simulink model "IEEE14_case"  (R2024b)
settings: Solver=FixedStepAuto  StartTime=0  StopTime=2  FixedStep=1e-7  RelTol=1e-3
values from neighbouring files (symbols this model uses):
  GFL_15_Bva = 0.009    [IEEE14_parameters.m]
  GFL_15_C_bus_pu = 7.179419    [IEEE14_parameters.m]
  GFL_15_f0 = 60    [IEEE14_parameters.m]
  GFL_15_I_id = 691.26967    [IEEE14_parameters.m]
  GFL_15_I_iq = 691.26967    [IEEE14_parameters.m]
  GFL_15_I_od = 45.2207    [IEEE14_parameters.m]
  GFL_15_I_oq = 45.2207    [IEEE14_parameters.m]
  GFL_15_I_pll = 0.78    [IEEE14_parameters.m]
  GFL_15_Kdi = 0.09    [IEEE14_parameters.m]
  GFL_15_Kdo = 0.9    [IEEE14_parameters.m]
  GFL_15_Kqi = 0.09    [IEEE14_parameters.m]
  GFL_15_Kqo = 0.9    [IEEE14_parameters.m]
  GFL_15_Lg_pu = 0.631447    [IEEE14_parameters.m]
  GFL_15_mode = 1    [IEEE14_parameters.m]
  GFL_15_P_id = 3.7166    [IEEE14_parameters.m]
  GFL_15_P_iq = 3.7166    [IEEE14_parameters.m]
  GFL_15_P_od = 0.4798    [IEEE14_parameters.m]
  GFL_15_P_oq = 0.4798    [IEEE14_parameters.m]
  GFL_15_P_pll = 290.42    [IEEE14_parameters.m]
  GFL_15_Qe_ref = 0.2    [IEEE14_parameters.m]
  GFL_15_Rg_pu = 0.024016    [IEEE14_parameters.m]
  GFL_15_Sbase = 1.000000e+4    (= 10000)    [IEEE14_parameters.m]
  GFL_15_Tdi = 0.01    [IEEE14_parameters.m]
  GFL_15_Tdo = 0.2    [IEEE14_parameters.m]
  GFL_15_Tqi = 0.01    [IEEE14_parameters.m]
  GFL_15_Tqo = 0.2    [IEEE14_parameters.m]
  GFL_15_Vbase = 380    [IEEE14_parameters.m]
  GFL_15_Vdc_ref = 1.011475    [IEEE14_parameters.m]
  GFL_15_Vdcbase = 700    [IEEE14_parameters.m]
  GFL_15_vq_ref = 0    [IEEE14_parameters.m]
  GFL_16_Bva = 0.002    [IEEE14_parameters.m]
  GFL_16_C_bus_pu = 7.179419    [IEEE14_parameters.m]
  GFL_16_f0 = 60    [IEEE14_parameters.m]
  GFL_16_I_id = 691.26967    [IEEE14_parameters.m]
  GFL_16_I_iq = 691.26967    [IEEE14_parameters.m]
  GFL_16_I_od = 45.2207    [IEEE14_parameters.m]
  GFL_16_I_oq = 45.2207    [IEEE14_parameters.m]
  GFL_16_I_pll = 0.78    [IEEE14_parameters.m]
  GFL_16_Kdi = 0.05    [IEEE14_parameters.m]
  GFL_16_Kdo = 0.5    [IEEE14_parameters.m]
  GFL_16_Kqi = 0.05    [IEEE14_parameters.m]
  GFL_16_Kqo = 0.5    [IEEE14_parameters.m]
  GFL_16_Lg_pu = 0.631447    [IEEE14_parameters.m]
  GFL_16_mode = 1    [IEEE14_parameters.m]
  GFL_16_P_id = 3.7166    [IEEE14_parameters.m]
  GFL_16_P_iq = 3.7166    [IEEE14_parameters.m]
  GFL_16_P_od = 0.4798    [IEEE14_parameters.m]
  GFL_16_P_oq = 0.4798    [IEEE14_parameters.m]
  GFL_16_P_pll = 290.42    [IEEE14_parameters.m]
  GFL_16_Qe_ref = 0.2    [IEEE14_parameters.m]
  GFL_16_Rg_pu = 0.024016    [IEEE14_parameters.m]
  GFL_16_Sbase = 1.000000e+4    (= 10000)    [IEEE14_parameters.m]
  GFL_16_Tdi = 0.01    [IEEE14_parameters.m]
  GFL_16_Tdo = 0.2    [IEEE14_parameters.m]
  GFL_16_Tqi = 0.01    [IEEE14_parameters.m]
  GFL_16_Tqo = 0.2    [IEEE14_parameters.m]
  GFL_16_Vbase = 380    [IEEE14_parameters.m]
  GFL_16_Vdc_ref = 1.01144    [IEEE14_parameters.m]
  GFL_16_Vdcbase = 700    [IEEE14_parameters.m]
  GFL_16_vq_ref = 0    [IEEE14_parameters.m]
  GFL_17_Bva = 0.002    [IEEE14_parameters.m]
  GFL_17_C_bus_pu = 7.179419    [IEEE14_parameters.m]
  GFL_17_f0 = 60    [IEEE14_parameters.m]
  GFL_17_I_id = 691.26967    [IEEE14_parameters.m]
  GFL_17_I_iq = 691.26967    [IEEE14_parameters.m]
  GFL_17_I_od = 45.2207    [IEEE14_parameters.m]
  GFL_17_I_oq = 45.2207    [IEEE14_parameters.m]
  GFL_17_I_pll = 0.78    [IEEE14_parameters.m]
  GFL_17_Kdi = 0.05    [IEEE14_parameters.m]
  GFL_17_Kdo = 0.5    [IEEE14_parameters.m]
  GFL_17_Kqi = 0.05    [IEEE14_parameters.m]
  GFL_17_Kqo = 0.5    [IEEE14_parameters.m]
  GFL_17_Lg_pu = 0.631447    [IEEE14_parameters.m]
  GFL_17_mode = 1    [IEEE14_parameters.m]
  GFL_17_P_id = 3.7166    [IEEE14_parameters.m]
  GFL_17_P_iq = 3.7166    [IEEE14_parameters.m]
  GFL_17_P_od = 0.4798    [IEEE14_parameters.m]
  GFL_17_P_oq = 0.4798    [IEEE14_parameters.m]
  GFL_17_P_pll = 290.42    [IEEE14_parameters.m]
  GFL_17_Qe_ref = 0.2    [IEEE14_parameters.m]
  GFL_17_Rg_pu = 0.024016    [IEEE14_parameters.m]
  GFL_17_Sbase = 1.000000e+4    (= 10000)    [IEEE14_parameters.m]
  GFL_17_Tdi = 0.01    [IEEE14_parameters.m]
  GFL_17_Tdo = 0.2    [IEEE14_parameters.m]
  GFL_17_Tqi = 0.01    [IEEE14_parameters.m]
  GFL_17_Tqo = 0.2    [IEEE14_parameters.m]
  GFL_17_Vbase = 380    [IEEE14_parameters.m]
  GFL_17_Vdc_ref = 1.011632    [IEEE14_parameters.m]
  GFL_17_Vdcbase = 700    [IEEE14_parameters.m]
  GFL_17_vq_ref = 0    [IEEE14_parameters.m]
  GFL_18_Bva = 0.002    [IEEE14_parameters.m]
  GFL_18_C_bus_pu = 7.179419    [IEEE14_parameters.m]
  GFL_18_f0 = 60    [IEEE14_parameters.m]
  GFL_18_I_id = 691.26967    [IEEE14_parameters.m]
  GFL_18_I_iq = 691.26967    [IEEE14_parameters.m]
  GFL_18_I_od = 45.2207    [IEEE14_parameters.m]
  GFL_18_I_oq = 45.2207    [IEEE14_parameters.m]
  GFL_18_I_pll = 0.78    [IEEE14_parameters.m]
  GFL_18_Kdi = 0.05    [IEEE14_parameters.m]
  GFL_18_Kdo = 0.5    [IEEE14_parameters.m]
  GFL_18_Kqi = 0.05    [IEEE14_parameters.m]
  GFL_18_Kqo = 0.5    [IEEE14_parameters.m]
  GFL_18_Lg_pu = 0.631447    [IEEE14_parameters.m]
  GFL_18_mode = 1    [IEEE14_parameters.m]
  GFL_18_P_id = 3.7166    [IEEE14_parameters.m]
  GFL_18_P_iq = 3.7166    [IEEE14_parameters.m]
  GFL_18_P_od = 0.4798    [IEEE14_parameters.m]
  GFL_18_P_oq = 0.4798    [IEEE14_parameters.m]
  GFL_18_P_pll = 290.42    [IEEE14_parameters.m]
  GFL_18_Qe_ref = 0.2    [IEEE14_parameters.m]
  GFL_18_Rg_pu = 0.024016    [IEEE14_parameters.m]
  GFL_18_Sbase = 1.000000e+4    (= 10000)    [IEEE14_parameters.m]
  GFL_18_Tdi = 0.01    [IEEE14_parameters.m]
  GFL_18_Tdo = 0.2    [IEEE14_parameters.m]
  GFL_18_Tqi = 0.01    [IEEE14_parameters.m]
  GFL_18_Tqo = 0.2    [IEEE14_parameters.m]
  GFL_18_Vbase = 380    [IEEE14_parameters.m]
  GFL_18_Vdc_ref = 1.011572    [IEEE14_parameters.m]
  GFL_18_Vdcbase = 700    [IEEE14_parameters.m]
  GFL_18_vq_ref = 0    [IEEE14_parameters.m]
  ... (+180 more)
(part 11 of 25)

== system IEEE14_case/GFL_16/d_Phi_gb_GFL_16_block ==
  note: d_Phi_gb_GFL_16 in case14gfl
      | $I_{\mathrm{id}}\,\left(\mathrm{Idv}_{\mathrm{GFL},16}+\Phi _{\mathrm{ga},\mathrm{GFL},16}-i_{\mathrm{gd},\mathrm{GFL},16}+P_{\mathrm{od}}\,\left(V_{\mathrm{dc},\mathrm{GFL},16}-\mathrm{Vdcbase}\,\mathrm{Vdc}_{\mathrm{ref}}\right)-\mathrm{Bva}\,\mathrm{Vbase}\,\left(v_{d,\mathrm{GFL},16}\,\cos\left(\theta _{\mathrm{pll},\mathrm{GFL},16}\right)-v_{q,\mathrm{GFL},16}\,\sin\left(\theta _{\mathrm{pll},\mathrm{GFL},16}\right)\right)\right)$
      | Automatically generated on 2025-10-09 21:36:07 .
  Input_v_d_GFL_16_5796c : Inport
  State_theta_pll_GFL_16_9faca : Inport  Port=2
  Input_v_q_GFL_16_58470 : Inport  Port=3
  State_theta_pll_GFL_16_1f0e5 : Inport  Port=4
  State_Idv_GFL_16_00ce2 : Inport  Port=5
  State_V_dc_GFL_16_186eb : Inport  Port=6
  State_Phi_ga_GFL_16_9aa12 : Inport  Port=7
  State_i_gd_GFL_16_104f5 : Inport  Port=8
  Add_816d2 : Sum
  Add_8c69a : Sum
  Add_ee524 : Sum
  Constant_-1_c479b : Constant  Value=-1
  Constant_Bva_cc442 : Constant  Value=Bva
  Constant_I_id_7e45e : Constant  Value=I_id
  Constant_P_od_57961 : Constant  Value=P_od
  Constant_Vbase_d7372 : Constant  Value=Vbase
  Constant_Vdc_ref_5c322 : Constant  Value=Vdc_ref
  Constant_Vdcbase_67ddd : Constant  Value=Vdcbase
  MathFunc_cos_ca6bf : Trigonometry  Operator=cos
  MathFunc_sin_e0267 : Trigonometry
  Product_2926b : Product
  Product_2d34a : Product
  Product_4ef76 : Product
  Product_59aab : Product
  Product_6212c : Product
  Product_b48db : Product
  Product_c4ab1 : Product
  Product_e24fb : Product
  Subtract_1bdde : Sum  Inputs=+-
  Subtract_e3d0d : Sum  Inputs=+-
  Subtract_eb397 : Sum  Inputs=+-
  Blockout_d_Phi_gb_GFL_16_e3dc3 : Outport
  wires:
  State_theta_pll_GFL_16_9faca/1 -> MathFunc_cos_ca6bf/1
  Constant_Bva_cc442/1 -> Product_c4ab1/2
  State_theta_pll_GFL_16_1f0e5/1 -> MathFunc_sin_e0267/1
  Product_c4ab1/1 -> Product_2d34a/1
  Constant_-1_c479b/1 -> Product_c4ab1/1
  Input_v_d_GFL_16_5796c/1 -> Product_59aab/1
  MathFunc_cos_ca6bf/1 -> Product_59aab/2
  Product_b48db/1 -> Subtract_1bdde/2
  Input_v_q_GFL_16_58470/1 -> Product_b48db/1
  MathFunc_sin_e0267/1 -> Product_b48db/2
  Constant_Vbase_d7372/1 -> Product_2d34a/2
  Product_59aab/1 -> Subtract_1bdde/1
  State_Phi_ga_GFL_16_9aa12/1 -> Add_816d2/2
  Constant_Vdc_ref_5c322/1 -> Product_4ef76/1
  Constant_Vdcbase_67ddd/1 -> Product_4ef76/2
  Product_2d34a/1 -> Product_e24fb/1
  Subtract_1bdde/1 -> Product_e24fb/2
  State_i_gd_GFL_16_104f5/1 -> Subtract_e3d0d/2
  State_V_dc_GFL_16_186eb/1 -> Subtract_eb397/1
  Product_4ef76/1 -> Subtract_eb397/2
  Product_e24fb/1 -> Add_8c69a/1
  State_Idv_GFL_16_00ce2/1 -> Add_8c69a/2
  Product_2926b/1 -> Add_ee524/2
  Constant_P_od_57961/1 -> Product_2926b/1
  Subtract_eb397/1 -> Product_2926b/2
  Add_8c69a/1 -> Add_ee524/1
  Add_ee524/1 -> Add_816d2/1
  Add_816d2/1 -> Subtract_e3d0d/1
  Constant_I_id_7e45e/1 -> Product_6212c/1
  Subtract_e3d0d/1 -> Product_6212c/2
  Product_6212c/1 -> Blockout_d_Phi_gb_GFL_16_e3dc3/1

== system IEEE14_case/GFL_16/d_Phi_gc_GFL_16_block ==
  note: d_Phi_gc_GFL_16 in case14gfl
      | $-I_{\mathrm{oq}}\,\left(\mathrm{Qe}_{\mathrm{ref}}\,\mathrm{Sbase}+1.73205080756888\,\mathrm{Vbase}\,i_{\mathrm{gd},\mathrm{GFL},16}\,\left(v_{q,\mathrm{GFL},16}\,\cos\left(\theta _{\mathrm{pll},\mathrm{GFL},16}\right)+v_{d,\mathrm{GFL},16}\,\sin\left(\theta _{\mathrm{pll},\mathrm{GFL},16}\right)\right)+1.73205080756888\,\mathrm{Vbase}\,i_{\mathrm{gq},\mathrm{GFL},16}\,\left(v_{d,\mathrm{GFL},16}\,\cos\left(\theta _{\mathrm{pll},\mathrm{GFL},16}\right)-v_{q,\mathrm{GFL},16}\,\sin\left(\theta _{\mathrm{pll},\mathrm{GFL},16}\right)\right)\right)$
      | Automatically generated on 2025-10-09 21:36:09 .
  State_i_gd_GFL_16_f5bc3 : Inport
  Input_v_d_GFL_16_5298e : Inport  Port=2
  State_theta_pll_GFL_16_2a2ae : Inport  Port=3
  Input_v_q_GFL_16_b8cf3 : Inport  Port=4
  State_theta_pll_GFL_16_9a1c0 : Inport  Port=5
  State_i_gq_GFL_16_12809 : Inport  Port=6
  Input_v_d_GFL_16_c77ca : Inport  Port=7
  State_theta_pll_GFL_16_c56ef : Inport  Port=8
  Input_v_q_GFL_16_61e16 : Inport  Port=9
  State_theta_pll_GFL_16_a6854 : Inport  Port=10
  Add_9f244 : Sum
  Constant_-1_d068e : Constant  Value=-1
  Constant_1.73205080756888_1ab3f : Constant  Value=1.73205080756888
  Constant_1.73205080756888_3e260 : Constant  Value=1.73205080756888
  Constant_I_oq_16e38 : Constant  Value=I_oq
  Constant_Qe_ref_4cc63 : Constant  Value=Qe_ref
  Constant_Sbase_67194 : Constant  Value=Sbase
  Constant_Vbase_67024 : Constant  Value=Vbase
  Constant_Vbase_c2ada : Constant  Value=Vbase
  MathFunc_cos_8d063 : Trigonometry  Operator=cos
  MathFunc_cos_e387c : Trigonometry  Operator=cos
  MathFunc_sin_1c9af : Trigonometry
  MathFunc_sin_fc0e6 : Trigonometry
  Product_1eb07 : Product
  Product_2f77b : Product
  Product_396d7 : Product
  Product_4fce4 : Product
  Product_59751 : Product
  Product_6bdde : Product
  Product_70e4a : Product
  Product_73ed6 : Product
  Product_b9821 : Product
  Product_c0659 : Product
  Product_e5fa5 : Product
  Product_ed71a : Product
  Product_f25bb : Product
  Subtract_08a0b : Sum  Inputs=+-
  Subtract_bd4c9 : Sum  Inputs=+-
  Subtract_ee10c : Sum  Inputs=+-
  Blockout_d_Phi_gc_GFL_16_21552 : Outport
  wires:
  Product_c0659/1 -> Product_2f77b/1
  Constant_Vbase_c2ada/1 -> Product_4fce4/2
  State_theta_pll_GFL_16_2a2ae/1 -> MathFunc_sin_1c9af/1
  State_theta_pll_GFL_16_9a1c0/1 -> MathFunc_cos_e387c/1
  MathFunc_cos_e387c/1 -> Product_b9821/2
  Product_4fce4/1 -> Product_c0659/1
  Constant_1.73205080756888_3e260/1 -> Product_4fce4/1
  Product_e5fa5/1 -> Add_9f244/1
  Input_v_d_GFL_16_5298e/1 -> Product_e5fa5/1
  MathFunc_sin_1c9af/1 -> Product_e5fa5/2
  Product_b9821/1 -> Add_9f244/2
  Input_v_q_GFL_16_b8cf3/1 -> Product_b9821/1
  MathFunc_cos_8d063/1 -> Product_59751/2
  State_theta_pll_GFL_16_c56ef/1 -> MathFunc_cos_8d063/1
  MathFunc_sin_fc0e6/1 -> Product_f25bb/2
  State_theta_pll_GFL_16_a6854/1 -> MathFunc_sin_fc0e6/1
  Constant_-1_d068e/1 -> Product_1eb07/1
  Product_2f77b/1 -> Subtract_bd4c9/2
  Constant_Qe_ref_4cc63/1 -> Product_1eb07/2
  State_i_gd_GFL_16_f5bc3/1 -> Product_c0659/2
  Product_396d7/1 -> Product_6bdde/1
  Constant_1.73205080756888_1ab3f/1 -> Product_396d7/1
  Product_6bdde/1 -> Product_73ed6/1
  Constant_Vbase_67024/1 -> Product_396d7/2
  Product_59751/1 -> Subtract_08a0b/1
  Product_1eb07/1 -> Product_70e4a/1
  Input_v_d_GFL_16_c77ca/1 -> Product_59751/1
  Input_v_q_GFL_16_61e16/1 -> Product_f25bb/1
  Constant_Sbase_67194/1 -> Product_70e4a/2
  Add_9f244/1 -> Product_2f77b/2
  Constant_I_oq_16e38/1 -> Product_ed71a/1
  State_i_gq_GFL_16_12809/1 -> Product_6bdde/2
  Product_f25bb/1 -> Subtract_08a0b/2
  Product_70e4a/1 -> Subtract_bd4c9/1
  Subtract_08a0b/1 -> Product_73ed6/2
  Subtract_bd4c9/1 -> Subtract_ee10c/1
  Product_73ed6/1 -> Subtract_ee10c/2
  Subtract_ee10c/1 -> Product_ed71a/2
  Product_ed71a/1 -> Blockout_d_Phi_gc_GFL_16_21552/1

== system IEEE14_case/GFL_16/d_Phi_gd_GFL_16_block ==
  note: d_Phi_gd_GFL_16 in case14gfl
      | $I_{\mathrm{iq}}\,\left(\mathrm{Iqv}_{\mathrm{GFL},16}+\Phi _{\mathrm{gc},\mathrm{GFL},16}-i_{\mathrm{gq},\mathrm{GFL},16}-P_{\mathrm{oq}}\,\left(\mathrm{Qe}_{\mathrm{ref}}\,\mathrm{Sbase}+1.73205080756888\,\mathrm{Vbase}\,i_{\mathrm{gd},\mathrm{GFL},16}\,\left(v_{q,\mathrm{GFL},16}\,\cos\left(\theta _{\mathrm{pll},\mathrm{GFL},16}\right)+v_{d,\mathrm{GFL},16}\,\sin\left(\theta _{\mathrm{pll},\mathrm{GFL},16}\right)\right)+1.73205080756888\,\mathrm{Vbase}\,i_{\mathrm{gq},\mathrm{GFL},16}\,\left(v_{d,\mathrm{GFL},16}\,\cos\left(\theta _{\mathrm{pll},\mathrm{GFL},16}\right)-v_{q,\mathrm{GFL},16}\,\sin\left(\theta _{\mathrm{pll},\mathrm{GFL},16}\right)\right)\right)+\mathrm{Bva}\,\mathrm{Vbase}\,\left(v_{q,\mathrm{GFL},16}\,\cos\left(\theta _{\mathrm{pll},\mathrm{GFL},16}\right)+v_{d,\mathrm{GFL},16}\,\sin\left(\theta _{\mathrm{pll},\mathrm{GFL},16}\right)\right)\right)$
      | Automatically generated on 2025-10-09 21:36:13 .
  Input_v_d_GFL_16_9b711 : Inport
  State_theta_pll_GFL_16_648b2 : Inport  Port=2
  Input_v_q_GFL_16_c9e4f : Inport  Port=3
  State_theta_pll_GFL_16_e1421 : Inport  Port=4
  State_Iqv_GFL_16_6ee1c : Inport  Port=5
  State_i_gd_GFL_16_6aeee : Inport  Port=6
  Input_v_d_GFL_16_a7f85 : Inport  Port=7
  State_theta_pll_GFL_16_9c942 : Inport  Port=8
  Input_v_q_GFL_16_d5137 : Inport  Port=9
  State_theta_pll_GFL_16_5c378 : Inport  Port=10
  State_i_gq_GFL_16_a69ee : Inport  Port=11
  Input_v_d_GFL_16_1cbf7 : Inport  Port=12
  State_theta_pll_GFL_16_6f123 : Inport  Port=13
  Input_v_q_GFL_16_69c8c : Inport  Port=14
  State_theta_pll_GFL_16_ebd89 : Inport  Port=15
  State_Phi_gc_GFL_16_a3666 : Inport  Port=16
  State_i_gq_GFL_16_a143d : Inport  Port=17
  Add_25052 : Sum
  Add_4ccd0 : Sum
  Add_8848f : Sum
  Add_ca996 : Sum
  Add_ec70f : Sum
  Constant_-1_88cd8 : Constant  Value=-1
  Constant_1.73205080756888_3396c : Constant  Value=1.73205080756888
  Constant_1.73205080756888_d617b : Constant  Value=1.73205080756888
  Constant_Bva_7e4b7 : Constant  Value=Bva
  Constant_I_iq_112b7 : Constant  Value=I_iq
  Constant_P_oq_4cce5 : Constant  Value=P_oq
  Constant_Qe_ref_93a57 : Constant  Value=Qe_ref
  Constant_Sbase_e2cd0 : Constant  Value=Sbase
  Constant_Vbase_039f5 : Constant  Value=Vbase
  Constant_Vbase_a3316 : Constant  Value=Vbase
  Constant_Vbase_be2b5 : Constant  Value=Vbase
  MathFunc_cos_518fc : Trigonometry  Operator=cos
  MathFunc_cos_a487e : Trigonometry  Operator=cos
  MathFunc_cos_c3736 : Trigonometry  Operator=cos
  MathFunc_sin_243eb : Trigonometry
  MathFunc_sin_a3588 : Trigonometry
  MathFunc_sin_bcd20 : Trigonometry
  Product_02c56 : Product
  Product_09f61 : Product
  Product_110c1 : Product
  Product_225ea : Product
  Product_2c3a6 : Product
  Product_2e02e : Product
  Product_3a99f : Product
  Product_43745 : Product
  Product_4da1f : Product
  Product_4e7c3 : Product
  Product_795ee : Product
  Product_7b424 : Product
  Product_7dc20 : Product
  Product_a6212 : Product
  Product_aac61 : Product
  Product_bbe8c : Product
  Product_c7878 : Product
  Product_e0150 : Product
  Subtract_13f81 : Sum  Inputs=+-
  Subtract_6cb63 : Sum  Inputs=+-
  Subtract_7336c : Sum  Inputs=+-
  Subtract_acad4 : Sum  Inputs=+-
  Blockout_d_Phi_gd_GFL_16_8a731 : Outport
  wires:
  State_theta_pll_GFL_16_9c942/1 -> MathFunc_sin_243eb/1
  MathFunc_sin_243eb/1 -> Product_225ea/2
  Product_7b424/1 -> Product_43745/1
  Constant_Vbase_be2b5/1 -> Product_110c1/2
  State_theta_pll_GFL_16_5c378/1 -> MathFunc_cos_a487e/1
  Constant_1.73205080756888_3396c/1 -> Product_110c1/1
  Constant_Qe_ref_93a57/1 -> Product_a6212/2
  Input_v_d_GFL_16_a7f85/1 -> Product_225ea/1
  Input_v_q_GFL_16_d5137/1 -> Product_c7878/1
  MathFunc_cos_a487e/1 -> Product_c7878/2
  State_theta_pll_GFL_16_6f123/1 -> MathFunc_cos_c3736/1
  State_theta_pll_GFL_16_ebd89/1 -> MathFunc_sin_bcd20/1
  State_Iqv_GFL_16_6ee1c/1 -> Add_ec70f/2
  State_theta_pll_GFL_16_648b2/1 -> MathFunc_sin_a3588/1
  State_theta_pll_GFL_16_e1421/1 -> MathFunc_cos_518fc/1
  Constant_-1_88cd8/1 -> Product_a6212/1
  State_i_gd_GFL_16_6aeee/1 -> Product_7b424/2
  Product_110c1/1 -> Product_7b424/1
  Product_225ea/1 -> Add_8848f/1
  Product_3a99f/1 -> Add_ec70f/1
  Product_c7878/1 -> Add_8848f/2
  Constant_Bva_7e4b7/1 -> Product_4da1f/1
  Constant_1.73205080756888_d617b/1 -> Product_7dc20/1
  Add_ec70f/1 -> Add_4ccd0/1
  Product_7dc20/1 -> Product_2e02e/1
  Constant_Vbase_a3316/1 -> Product_7dc20/2
  Input_v_d_GFL_16_1cbf7/1 -> Product_aac61/1
  MathFunc_cos_c3736/1 -> Product_aac61/2
  Product_2c3a6/1 -> Subtract_acad4/2
  Input_v_q_GFL_16_69c8c/1 -> Product_2c3a6/1
  MathFunc_sin_bcd20/1 -> Product_2c3a6/2
  Input_v_d_GFL_16_9b711/1 -> Product_4e7c3/1
  Constant_I_iq_112b7/1 -> Product_795ee/1
  MathFunc_sin_a3588/1 -> Product_4e7c3/2
  Product_02c56/1 -> Add_25052/2
  Input_v_q_GFL_16_c9e4f/1 -> Product_02c56/1
  Product_795ee/1 -> Blockout_d_Phi_gd_GFL_16_8a731/1
  MathFunc_cos_518fc/1 -> Product_02c56/2
  Product_a6212/1 -> Product_bbe8c/1
  Constant_Sbase_e2cd0/1 -> Product_bbe8c/2
  Add_8848f/1 -> Product_43745/2
  State_i_gq_GFL_16_a69ee/1 -> Product_2e02e/2
  Add_ca996/1 -> Subtract_6cb63/1
  Product_aac61/1 -> Subtract_acad4/1
  Product_e0150/1 -> Add_4ccd0/2
  Constant_P_oq_4cce5/1 -> Product_e0150/1
  Constant_Vbase_039f5/1 -> Product_4da1f/2
  Product_4e7c3/1 -> Add_25052/1
  Subtract_6cb63/1 -> Product_795ee/2
  Product_bbe8c/1 -> Subtract_13f81/1
  Product_43745/1 -> Subtract_13f81/2
  Product_2e02e/1 -> Product_09f61/1
  Subtract_acad4/1 -> Product_09f61/2
  Product_4da1f/1 -> Product_3a99f/1
  Add_25052/1 -> Product_3a99f/2
  Subtract_13f81/1 -> Subtract_7336c/1
  Product_09f61/1 -> Subtract_7336c/2
  Add_4ccd0/1 -> Add_ca996/1
  Subtract_7336c/1 -> Product_e0150/2
  State_Phi_gc_GFL_16_a3666/1 -> Add_ca996/2
  State_i_gq_GFL_16_a143d/1 -> Subtract_6cb63/2

== system IEEE14_case/GFL_16/d_Phipll_GFL_16_block ==
  note: d_Phipll_GFL_16 in case14gfl
      | $-I_{\mathrm{pll}}\,\left(\mathrm{vq}_{\mathrm{ref}}+v_{q,\mathrm{GFL},16}\,\cos\left(\theta _{\mathrm{pll},\mathrm{GFL},16}\right)+v_{d,\mathrm{GFL},16}\,\sin\left(\theta _{\mathrm{pll},\mathrm{GFL},16}\right)\right)$
      | Automatically generated on 2025-10-09 21:36:04 .
  Input_v_d_GFL_16_4ce7f : Inport
  State_theta_pll_GFL_16_31350 : Inport  Port=2
  Input_v_q_GFL_16_4b778 : Inport  Port=3
  State_theta_pll_GFL_16_5a7c5 : Inport  Port=4
  Constant_-1_ec456 : Constant  Value=-1
  Constant_I_pll_64c72 : Constant  Value=I_pll
  Constant_vq_ref_5ee97 : Constant  Value=vq_ref
  MathFunc_cos_6b328 : Trigonometry  Operator=cos
  MathFunc_sin_778af : Trigonometry
  Product_09b53 : Product
  Product_82336 : Product
  Product_82c7a : Product
  Product_8b6c1 : Product
  Subtract_12c26 : Sum  Inputs=+-
  Subtract_5a5f5 : Sum  Inputs=+-
  Blockout_d_Phipll_GFL_16_c41f9 : Outport
  wires:
  Constant_-1_ec456/1 -> Product_82c7a/1
  Input_v_d_GFL_16_4ce7f/1 -> Product_82c7a/2
  Input_v_q_GFL_16_4b778/1 -> Product_09b53/1
  State_theta_pll_GFL_16_31350/1 -> MathFunc_sin_778af/1
  State_theta_pll_GFL_16_5a7c5/1 -> MathFunc_cos_6b328/1
  Product_82c7a/1 -> Product_82336/1
  MathFunc_sin_778af/1 -> Product_82336/2
  MathFunc_cos_6b328/1 -> Product_09b53/2
  Product_82336/1 -> Subtract_12c26/1
  Product_09b53/1 -> Subtract_12c26/2
  Subtract_12c26/1 -> Subtract_5a5f5/1
  Constant_vq_ref_5ee97/1 -> Subtract_5a5f5/2
  Constant_I_pll_64c72/1 -> Product_8b6c1/1
  Subtract_5a5f5/1 -> Product_8b6c1/2
  Product_8b6c1/1 -> Blockout_d_Phipll_GFL_16_c41f9/1

== system IEEE14_case/GFL_16/d_Psi_d_GFL_16_block ==
  note: d_Psi_d_GFL_16 in case14gfl
      | $-\frac{\Psi _{d,\mathrm{GFL},16}+\mathrm{Kdi}\,\mathrm{Vbase}\,\left(v_{q,\mathrm{GFL},16}\,\cos\left(\theta _{\mathrm{pll},\mathrm{GFL},16}\right)+v_{d,\mathrm{GFL},16}\,\sin\left(\theta _{\mathrm{pll},\mathrm{GFL},16}\right)\right)}{\mathrm{Tdi}}$
      | Automatically generated on 2025-10-09 21:36:15 .
  Input_v_d_GFL_16_6aa9b : Inport
  State_theta_pll_GFL_16_f203b : Inport  Port=2
  Input_v_q_GFL_16_54a29 : Inport  Port=3
  State_theta_pll_GFL_16_41daa : Inport  Port=4
  State_Psi_d_GFL_16_eadb2 : Inport  Port=5
  Add_3b283 : Sum
  Constant_-1_f90ab : Constant  Value=-1
  Constant_Kdi_e44a8 : Constant  Value=Kdi
  Constant_Tdi_e7c0a : Constant  Value=Tdi
  Constant_Vbase_bc0b3 : Constant  Value=Vbase
  Divide_594fb : Product  Inputs=*/
  MathFunc_cos_a6d89 : Trigonometry  Operator=cos
  MathFunc_sin_0b464 : Trigonometry
  Product_125bf : Product
  Product_255ec : Product
  Product_29218 : Product
  Product_7574a : Product
  Product_7fbe7 : Product
  Subtract_1436c : Sum  Inputs=+-
  Blockout_d_Psi_d_GFL_16_a9046 : Outport
  wires:
  State_theta_pll_GFL_16_f203b/1 -> MathFunc_sin_0b464/1
  Product_125bf/1 -> Product_255ec/1
  MathFunc_sin_0b464/1 -> Product_7574a/2
  State_theta_pll_GFL_16_41daa/1 -> MathFunc_cos_a6d89/1
  Constant_Kdi_e44a8/1 -> Product_125bf/2
  Constant_-1_f90ab/1 -> Product_125bf/1
  Input_v_d_GFL_16_6aa9b/1 -> Product_7574a/1
  MathFunc_cos_a6d89/1 -> Product_29218/2
  Input_v_q_GFL_16_54a29/1 -> Product_29218/1
  Constant_Vbase_bc0b3/1 -> Product_255ec/2
  Product_7574a/1 -> Add_3b283/1
  Product_29218/1 -> Add_3b283/2
  Constant_Tdi_e7c0a/1 -> Divide_594fb/2
  Product_255ec/1 -> Product_7fbe7/1
  Add_3b283/1 -> Product_7fbe7/2
  Product_7fbe7/1 -> Subtract_1436c/1
  State_Psi_d_GFL_16_eadb2/1 -> Subtract_1436c/2
  Subtract_1436c/1 -> Divide_594fb/1
  Divide_594fb/1 -> Blockout_d_Psi_d_GFL_16_a9046/1

== system IEEE14_case/GFL_16/d_Psi_q_GFL_16_block ==
  note: d_Psi_q_GFL_16 in case14gfl
      | $-\frac{\Psi _{q,\mathrm{GFL},16}-\mathrm{Kqi}\,\mathrm{Vbase}\,\left(v_{d,\mathrm{GFL},16}\,\cos\left(\theta _{\mathrm{pll},\mathrm{GFL},16}\right)-v_{q,\mathrm{GFL},16}\,\sin\left(\theta _{\mathrm{pll},\mathrm{GFL},16}\right)\right)}{\mathrm{Tqi}}$
      | Automatically generated on 2025-10-09 21:36:16 .
  Input_v_d_GFL_16_3fb89 : Inport
  State_theta_pll_GFL_16_b008b : Inport  Port=2
  Input_v_q_GFL_16_21710 : Inport  Port=3
  State_theta_pll_GFL_16_07f68 : Inport  Port=4
  State_Psi_q_GFL_16_7f6e6 : Inport  Port=5
  Constant_Kqi_2f792 : Constant  Value=Kqi
  Constant_Tqi_3eeb4 : Constant  Value=Tqi
  Constant_Vbase_7308a : Constant  Value=Vbase
  Divide_d9d39 : Product  Inputs=*/
  MathFunc_cos_fe187 : Trigonometry  Operator=cos
  MathFunc_sin_73dd1 : Trigonometry
  Product_6eff6 : Product
  Product_95516 : Product
  Product_dc201 : Product
  Product_f3afa : Product
  Subtract_36482 : Sum  Inputs=+-
  Subtract_a3d60 : Sum  Inputs=+-
  Blockout_d_Psi_q_GFL_16_c83e3 : Outport
  wires:
  Divide_d9d39/1 -> Blockout_d_Psi_q_GFL_16_c83e3/1
  State_theta_pll_GFL_16_b008b/1 -> MathFunc_cos_fe187/1
  State_theta_pll_GFL_16_07f68/1 -> MathFunc_sin_73dd1/1
  MathFunc_sin_73dd1/1 -> Product_dc201/2
  Product_95516/1 -> Subtract_a3d60/1
  Input_v_d_GFL_16_3fb89/1 -> Product_95516/1
  Constant_Kqi_2f792/1 -> Product_6eff6/1
  MathFunc_cos_fe187/1 -> Product_95516/2
  Product_dc201/1 -> Subtract_a3d60/2
  Input_v_q_GFL_16_21710/1 -> Product_dc201/1
  Constant_Vbase_7308a/1 -> Product_6eff6/2
  Product_6eff6/1 -> Product_f3afa/1
  Subtract_a3d60/1 -> Product_f3afa/2
  Product_f3afa/1 -> Subtract_36482/1
  State_Psi_q_GFL_16_7f6e6/1 -> Subtract_36482/2
  Subtract_36482/1 -> Divide_d9d39/1
  Constant_Tqi_3eeb4/1 -> Divide_d9d39/2

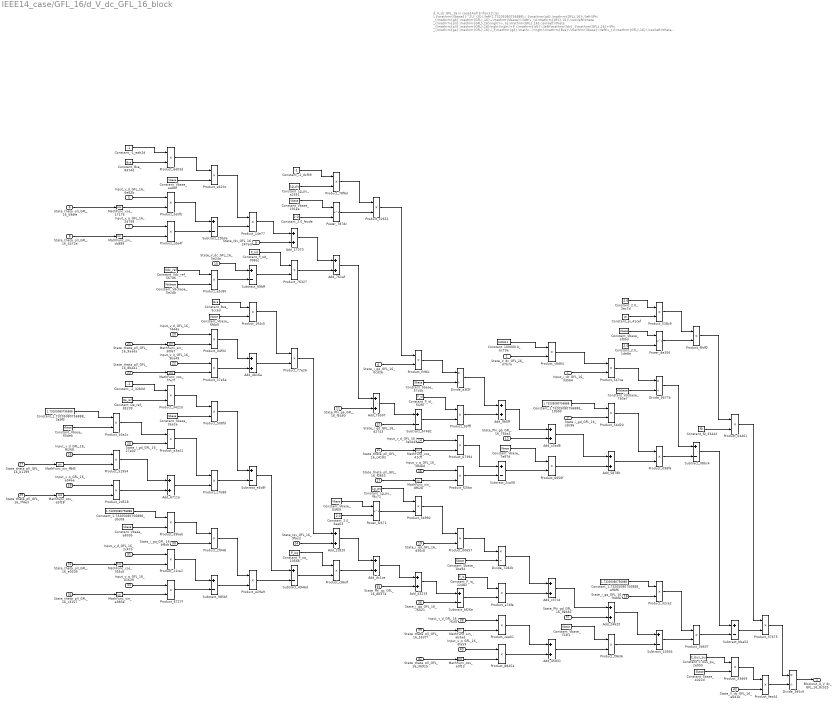
== system IEEE14_case/GFL_16/d_V_dc_GFL_16_block ==
  note: d_V_dc_GFL_16 in case14gfl
      | $-\frac{2\,\pi \,{\mathrm{Vbase}}^2\,f_{0}\,\left(1.73205080756888\,i_{\mathrm{gd},\mathrm{GFL},16}\,\left(\Phi _{\mathrm{gb},\mathrm{GFL},16}+\mathrm{Vbase}\,\left(v_{d,\mathrm{GFL},16}\,\cos\left(\theta _{\mathrm{pll},\mathrm{GFL},16}\right)-v_{q,\mathrm{GFL},16}\,\sin\left(\theta _{\mathrm{pll},\mathrm{GFL},16}\right)\right)+P_{\mathrm{id}}\,\left(\mathrm{Idv}_{\mathrm{GFL},16}+\Phi _{\mathrm{ga},\mathrm{GFL},16}-i_{\mathrm{gd},\mathrm{GFL},16}+P_{\mathrm{od}}\,\left(V_{\mathrm{dc},\mathrm{GFL},16}-\mathrm{Vdcbase}\,\mathrm{Vdc}_{\mathrm{ref}}\right)-\mathrm{Bva}\,\mathrm{Vbase}\,\left(v_{d,\mathrm{GFL},16}\,\cos\left(\theta _{\mathrm{pll},\mathrm{GFL},16}\right)-v_{q,\mathrm{GFL},16}\,\sin\left(\theta _{\mathrm{pll},\mathrm{GFL},16}\right)\right)\right)-\frac{\mathrm{Lg}_{\mathrm{pu}}\,{\mathrm{Vbase}}^2\,i_{\mathrm{gq},\mathrm{GFL},16}}{\mathrm{Sbase}}\right)+1.73205080756888\,i_{\mathrm{gq},\mathrm{GFL},16}\,\left(\Phi _{\mathrm{gd},\mathrm{GFL},16}-\mathrm{Vbase}\,\left(v_{q,\mathrm{GFL},16}\,\cos\left(\theta _{\mathrm{pll},\mathrm{GFL},16}\right)+v_{d,\mathrm{GFL},16}\,\sin\left(\theta _{\mathrm{pll},\mathrm{GFL},16}\right)\right)+P_{\mathrm{iq}}\,\left(\mathrm{Iqv}_{\mathrm{GFL},16}+\Phi _{\mathrm{gc},\mathrm{GFL},16}-i_{\mathrm{gq},\mathrm{GFL},16}-P_{\mathrm{oq}}\,\left(\mathrm{Qe}_{\mathrm{ref}}\,\mathrm{Sbase}+1.73205080756888\,\mathrm{Vbase}\,i_{\mathrm{gd},\mathrm{GFL},16}\,\left(v_{q,\mathrm{GFL},16}\,\cos\left(\theta _{\mathrm{pll},\mathrm{GFL},16}\right)+v_{d,\mathrm{GFL},16}\,\sin\left(\theta _{\mathrm{pll},\mathrm{GFL},16}\right)\right)+1.73205080756888\,\mathrm{Vbase}\,i_{\mathrm{gq},\mathrm{GFL},16}\,\left(v_{d,\mathrm{GFL},16}\,\cos\left(\theta _{\mathrm{pll},\mathrm{GFL},16}\right)-v_{q,\mathrm{GFL},16}\,\sin\left(\theta _{\mathrm{pll},\mathrm{GFL},16}\right)\right)\right)+\mathrm{Bva}\,\mathrm{Vbase}\,\left(v_{q,\mathrm{GFL},16}\,\cos\left(\theta _{\mathrm{pll},\mathrm{GFL},16}\right)+v_{d,\mathrm{GFL},16}\,\sin\left(\theta _{\mathrm{pll},\mathrm{GFL},16}\right)\right)\right)+\frac{\mathrm{Lg}_{\mathrm{pu}}\,{\mathrm{Vbase}}^2\,i_{\mathrm{gd},\mathrm{GFL},16}}{\mathrm{Sbase}}\right)-\frac{100000.0\,V_{\mathrm{dc},\mathrm{GFL},16}\,i_{\mathrm{dc},\mathrm{GFL},16}}{\mathrm{Vdcbase}}\right)}{C_{\mathrm{bus},\mathrm{pu}}\,\mathrm{Sbase}\,V_{\mathrm{dc},\mathrm{GFL},16}}$
      | Automatically generated on 2025-10-09 21:36:01 .
  State_V_dc_GFL_16_d7b7a : Inport
  Input_i_dc_GFL_16_33564 : Inport  Port=2
  State_i_gd_GFL_16_cdb96 : Inport  Port=3
  State_i_gq_GFL_16_0cd26 : Inport  Port=4
  Input_v_d_GFL_16_6e82b : Inport  Port=5
  State_theta_pll_GFL_16_59dfe : Inport  Port=6
  Input_v_q_GFL_16_2d758 : Inport  Port=7
  State_theta_pll_GFL_16_4472e : Inport  Port=8
  State_Idv_GFL_16_247ed : Inport  Port=9
  State_V_dc_GFL_16_5e24a : Inport  Port=10
  State_Phi_ga_GFL_16_f5490 : Inport  Port=11
  State_i_gd_GFL_16_d2743 : Inport  Port=12
  State_Phi_gb_GFL_16_76ba1 : Inport  Port=13
  Input_v_d_GFL_16_3e044 : Inport  Port=14
  State_theta_pll_GFL_16_c4182 : Inport  Port=15
  Input_v_q_GFL_16_384ed : Inport  Port=16
  State_theta_pll_GFL_16_f0853 : Inport  Port=17
  State_i_gq_GFL_16_94bfe : Inport  Port=18
  State_i_gd_GFL_16_d36c8 : Inport  Port=19
  Input_v_d_GFL_16_7444a : Inport  Port=20
  State_theta_pll_GFL_16_9aada : Inport  Port=21
  Input_v_q_GFL_16_9ba49 : Inport  Port=22
  State_theta_pll_GFL_16_8b441 : Inport  Port=23
  State_Iqv_GFL_16_9facd : Inport  Port=24
  State_i_gd_GFL_16_27e02 : Inport  Port=25
  Input_v_d_GFL_16_f6268 : Inport  Port=26
  State_theta_pll_GFL_16_b1199 : Inport  Port=27
  Input_v_q_GFL_16_a04ae : Inport  Port=28
  State_theta_pll_GFL_16_7f4e3 : Inport  Port=29
  State_i_gq_GFL_16_bf6cb : Inport  Port=30
  Input_v_d_GFL_16_2c47b : Inport  Port=31
  State_theta_pll_GFL_16_e0209 : Inport  Port=32
  Input_v_q_GFL_16_01629 : Inport  Port=33
  State_theta_pll_GFL_16_c3157 : Inport  Port=34
  State_Phi_gc_GFL_16_8b374 : Inport  Port=35
  State_i_gq_GFL_16_76021 : Inport  Port=36
  State_Phi_gd_GFL_16_9eb81 : Inport  Port=37
  Input_v_d_GFL_16_7f1f3 : Inport  Port=38
  State_theta_pll_GFL_16_5537f : Inport  Port=39
  Input_v_q_GFL_16_dfa59 : Inport  Port=40
  State_theta_pll_GFL_16_36915 : Inport  Port=41
  State_V_dc_GFL_16_a6d1b : Inport  Port=42
  Add_{17370,24620,43219,45831} (4 alike) : Sum
  Add_2c820 : Sum
  Add_4b16a : Sum
  Add_5878b : Sum
  Add_6711a : Sum
  Add_761ef : Sum
  Add_7ab97 : Sum
  Add_9b5ff : Sum
  Add_c37c4 : Sum
  Add_c3ad8 : Sum
  Add_dc1ce : Sum
  Constant_-1_32b0d : Constant  Value=-1
  Constant_-1_dcf39 : Constant  Value=-1
  Constant_-1_eab2d : Constant  Value=-1
  Constant_1.73205080756888_19b90 : Constant  Value=1.73205080756888
  Constant_1.73205080756888_3a9f3 : Constant  Value=1.73205080756888
  Constant_1.73205080756888_dbc08 : Constant  Value=1.73205080756888
  Constant_1.73205080756888_e9bf6 : Constant  Value=1.73205080756888
  Constant_100000.0_bc73e : Constant  Value=100000.0
  Constant_2.0_1de8e : Constant  Value=2.0
  Constant_2.0_3aa63 : Constant  Value=2.0
  Constant_2.0_3ec7d : Constant  Value=2.0
  Constant_2.0_facde : Constant  Value=2.0
  Constant_Bva_3ccad : Constant  Value=Bva
  Constant_Bva_8474d : Constant  Value=Bva
  Constant_C_bus_pu_2e055 : Constant  Value=C_bus_pu
  Constant_Lg_pu_a2551 : Constant  Value=Lg_pu
  Constant_Lg_pu_f9c71 : Constant  Value=Lg_pu
  Constant_P_id_f32f0 : Constant  Value=P_id
  Constant_P_iq_12482 : Constant  Value=P_iq
  Constant_P_od_098ac : Constant  Value=P_od
  Constant_P_oq_105b8 : Constant  Value=P_oq
  Constant_Qe_ref_85239 : Constant  Value=Qe_ref
  Constant_Sbase_1be94 : Constant  Value=Sbase
  Constant_Sbase_3aa2e : Constant  Value=Sbase
  Constant_Sbase_4022d : Constant  Value=Sbase
  Constant_Sbase_57c5b : Constant  Value=Sbase
  Constant_Vbase_04f09 : Constant  Value=Vbase
  Constant_Vbase_191ea : Constant  Value=Vbase
  Constant_Vbase_65deb : Constant  Value=Vbase
  Constant_Vbase_6fda9 : Constant  Value=Vbase
  Constant_Vbase_7e87d : Constant  Value=Vbase
  Constant_Vbase_aa88f : Constant  Value=Vbase
  Constant_Vbase_af0bd : Constant  Value=Vbase
  Constant_Vbase_e833b : Constant  Value=Vbase
  Constant_Vbase_f13f1 : Constant  Value=Vbase
  Constant_Vdc_ref_567d6 : Constant  Value=Vdc_ref
  Constant_Vdcbase_5e2db : Constant  Value=Vdcbase
  Constant_Vdcbase_783e7 : Constant  Value=Vdcbase
  Constant_f0_33442 : Constant  Value=f0
  Constant_pi_41cef : Constant  Value=pi
  Divide_3d5c9 : Product  Inputs=*/
  Divide_7282b : Product  Inputs=*/
  Divide_9b77b : Product  Inputs=*/
  Divide_a3f2f : Product  Inputs=*/
  MathFunc_cos_17176 : Trigonometry  Operator=cos
  MathFunc_cos_355c5 : Trigonometry  Operator=cos
  MathFunc_cos_41cff : Trigonometry  Operator=cos
  MathFunc_cos_a0f13 : Trigonometry  Operator=cos
  MathFunc_cos_a5f28 : Trigonometry  Operator=cos
  MathFunc_cos_f7e7f : Trigonometry  Operator=cos
  MathFunc_sin_30f67 : Trigonometry
  MathFunc_sin_8f628 : Trigonometry
  MathFunc_sin_a983e : Trigonometry
  MathFunc_sin_ab3ad : Trigonometry
  MathFunc_sin_dc889 : Trigonometry
  MathFunc_sin_ffbf3 : Trigonometry
  Power_787dc : Math  Operator=pow
  Power_de356 : Math  Operator=pow
  Power_f2671 : Math  Operator=pow
  Product_00657 : Product
  Product_04461 : Product
  Product_04f32 : Product
  Product_096f6 : Product
  Product_11ca1 : Product
  Product_14e77 : Product
  Product_164c5 : Product
  Product_2d518 : Product
  Product_2f948 : Product
  Product_32ca2 : Product
  Product_33d69 : Product
  Product_{34210,37675,51954,54992,67394,76327,88454} (7 alike) : Product
  Product_37e5e : Product
  Product_39beb : Product
  Product_3b637 : Product
  Product_429a9 : Product
  Product_508fd : Product
  Product_538c9 : Product
  Product_547ce : Product
  Product_54d20 : Product
  Product_6656f : Product
  Product_6727f : Product
  Product_6d03d : Product
  Product_77e26 : Product
  Product_78f6d : Product
  Product_93fff : Product
  Product_a3a41 : Product
  Product_a7bfe : Product
  Product_b3a2c : Product
  Product_b3dfc : Product
  Product_c2651 : Product
  Product_c7b88 : Product
  Product_c863f : Product
  Product_c8d64 : Product
  Product_cae01 : Product
  Product_cde4f : Product
  Product_e5c80 : Product
  Product_e623c : Product
  Product_f25ba : Product
  Product_f9636 : Product
  Product_f9df0 : Product
  Product_fc96c : Product
  Product_fea44 : Product
  Subtract_08bc4 : Sum  Inputs=+-
  Subtract_29b3a : Sum  Inputs=+-
  Subtract_2ca08 : Sum  Inputs=+-
  Subtract_43564 : Sum  Inputs=+-
  Subtract_4946d : Sum  Inputs=+-
  Subtract_67482 : Sum  Inputs=+-
  Subtract_89bff : Sum  Inputs=+-
  Subtract_985bf : Sum  Inputs=+-
  Subtract_bba52 : Sum  Inputs=+-
  Subtract_bf26e : Sum  Inputs=+-
  Subtract_e5c8f : Sum  Inputs=+-
  Blockout_d_V_dc_GFL_16_8cb25 : Outport
  wires:
  Product_f9df0/1 -> Product_04461/1
  State_i_gq_GFL_16_76021/1 -> Subtract_bf26e/2
  Product_88454/1 -> Add_45831/2
  Constant_Sbase_57c5b/1 -> Divide_a3f2f/2
  Product_6d03d/1 -> Product_e623c/1
  Input_v_q_GFL_16_a04ae/1 -> Product_2d518/1
  Constant_-1_32b0d/1 -> Product_34210/1
  Subtract_bba52/1 -> Product_37675/2
  Product_538c9/1 -> Product_f9df0/1
  Product_c863f/1 -> Add_dc1ce/2
  State_V_dc_GFL_16_a6d1b/1 -> Product_fea44/2
  Add_45831/1 -> Product_f9636/2
  Product_fea44/1 -> Divide_3d5c9/2
  Product_508fd/1 -> Subtract_e5c8f/1
  Product_6727f/1 -> Subtract_985bf/2
  Product_c2651/1 -> Product_fc96c/1
  MathFunc_cos_355c5/1 -> Product_11ca1/2
  Constant_Vbase_65deb/1 -> Product_b3a2c/2
  State_theta_pll_GFL_16_e0209/1 -> MathFunc_cos_355c5/1
  Add_c37c4/1 -> Add_24620/1
  Constant_1.73205080756888_19b90/1 -> Product_54d20/1
  Product_3b637/1 -> Subtract_bba52/2
  Divide_3d5c9/1 -> Blockout_d_V_dc_GFL_16_8cb25/1
  Constant_1.73205080756888_3a9f3/1 -> Product_b3a2c/1
  Product_547ce/1 -> Divide_9b77b/1
  Product_b3a2c/1 -> Product_a3a41/1
  Constant_C_bus_pu_2e055/1 -> Product_33d69/1
  Product_33d69/1 -> Product_fea44/1
  State_Phi_gd_GFL_16_9eb81/1 -> Add_24620/2
  Subtract_4946d/1 -> Product_c863f/2
  State_theta_pll_GFL_16_5537f/1 -> MathFunc_sin_ab3ad/1
  MathFunc_sin_ab3ad/1 -> Product_cae01/2
  Constant_Sbase_4022d/1 -> Product_33d69/2
  Add_24620/1 -> Subtract_43564/1
  Constant_pi_41cef/1 -> Product_538c9/2
  Input_v_d_GFL_16_2c47b/1 -> Product_11ca1/1
  Subtract_985bf/1 -> Product_429a9/2
  Add_5878b/1 -> Product_096f6/2
  Product_37675/1 -> Divide_3d5c9/1
  State_theta_pll_GFL_16_c4182/1 -> MathFunc_cos_41cff/1
  MathFunc_sin_30f67/1 -> Product_04f32/2
  State_Phi_gb_GFL_16_76ba1/1 -> Add_c3ad8/2
  State_i_gd_GFL_16_27e02/1 -> Product_a3a41/2
  Divide_7282b/1 -> Add_c37c4/1
  State_i_gq_GFL_16_94bfe/1 -> Product_32ca2/2
  Product_51954/1 -> Add_6711a/1
  Constant_Vbase_7e87d/1 -> Product_6656f/1
  Input_v_d_GFL_16_f6268/1 -> Product_51954/1
  Product_e5c80/1 -> Subtract_89bff/2
  Add_c3ad8/1 -> Add_5878b/1
  Subtract_43564/1 -> Product_3b637/2
  Product_c7b88/1 -> Subtract_e5c8f/2
  Add_43219/1 -> Subtract_bf26e/1
  Product_f9636/1 -> Subtract_43564/2
  State_Phi_gc_GFL_16_8b374/1 -> Add_43219/2
  MathFunc_cos_a0f13/1 -> Product_88454/2
  State_theta_pll_GFL_16_36915/1 -> MathFunc_cos_a0f13/1
  Product_f25ba/1 -> Subtract_2ca08/2
  MathFunc_cos_a5f28/1 -> Product_2d518/2
  Input_v_q_GFL_16_01629/1 -> Product_6727f/1
  Product_cae01/1 -> Add_45831/1
  Input_v_d_GFL_16_7f1f3/1 -> Product_cae01/1
  Product_04f32/1 -> Add_4b16a/1
  Input_v_q_GFL_16_dfa59/1 -> Product_88454/1
  Constant_Vdc_ref_567d6/1 -> Product_e5c80/1
  Power_787dc/1 -> Product_c2651/2
  Subtract_67482/1 -> Product_93fff/2
  Add_dc1ce/1 -> Add_43219/1
  Constant_Vbase_f13f1/1 -> Product_f9636/1
  State_i_gq_GFL_16_bf6cb/1 -> Product_2f948/2
  Product_a7bfe/1 -> Add_c37c4/2
  Subtract_bf26e/1 -> Product_a7bfe/2
  Constant_Qe_ref_85239/1 -> Product_34210/2
  State_theta_pll_GFL_16_f0853/1 -> MathFunc_sin_8f628/1
  Product_429a9/1 -> Subtract_4946d/2
  Input_v_d_GFL_16_3e044/1 -> Product_67394/1
  MathFunc_sin_ffbf3/1 -> Product_51954/2
  Constant_Vbase_e833b/1 -> Product_39beb/2
  MathFunc_sin_a983e/1 -> Product_6727f/2
  State_theta_pll_GFL_16_c3157/1 -> MathFunc_sin_a983e/1
  Product_11ca1/1 -> Subtract_985bf/1
  Product_2f948/1 -> Product_429a9/1
  Product_39beb/1 -> Product_2f948/1
  Constant_1.73205080756888_dbc08/1 -> Product_39beb/1
  Constant_2.0_1de8e/1 -> Power_de356/2
  Subtract_e5c8f/1 -> Subtract_4946d/1
  Product_6656f/1 -> Add_5878b/2
  Add_6711a/1 -> Product_c7b88/2
  Product_2d518/1 -> Add_6711a/2
  State_theta_pll_GFL_16_7f4e3/1 -> MathFunc_cos_a5f28/1
  Product_a3a41/1 -> Product_c7b88/1
  Product_67394/1 -> Subtract_2ca08/1
  State_theta_pll_GFL_16_b1199/1 -> MathFunc_sin_ffbf3/1
  Constant_Vbase_aa88f/1 -> Product_e623c/2
  Constant_Sbase_3aa2e/1 -> Product_508fd/2
  Product_34210/1 -> Product_508fd/1
  Constant_1.73205080756888_e9bf6/1 -> Product_32ca2/1
  Constant_P_oq_105b8/1 -> Product_c863f/1
  Add_7ab97/1 -> Subtract_67482/1
  Add_2c820/1 -> Add_dc1ce/1
  State_Iqv_GFL_16_9facd/1 -> Add_2c820/2
  Add_761ef/1 -> Add_7ab97/1
  Product_77e26/1 -> Add_2c820/1
  Add_4b16a/1 -> Product_77e26/2
  Product_37e5e/1 -> Add_4b16a/2
  State_i_gd_GFL_16_d2743/1 -> Subtract_67482/2
  MathFunc_cos_f7e7f/1 -> Product_37e5e/2
  State_theta_pll_GFL_16_8b441/1 -> MathFunc_cos_f7e7f/1
  MathFunc_cos_17176/1 -> Product_b3dfc/2
  Input_v_q_GFL_16_9ba49/1 -> Product_37e5e/1
  Product_164c5/1 -> Product_77e26/1
  Add_17370/1 -> Add_761ef/1
  State_theta_pll_GFL_16_9aada/1 -> MathFunc_sin_30f67/1
  Input_v_d_GFL_16_7444a/1 -> Product_04f32/1
  Constant_100000.0_bc73e/1 -> Product_c8d64/1
  Constant_Vbase_6fda9/1 -> Product_164c5/2
  Constant_Bva_3ccad/1 -> Product_164c5/1
  Constant_P_iq_12482/1 -> Product_a7bfe/1
  Product_e623c/1 -> Product_14e77/1
  Constant_Sbase_1be94/1 -> Divide_7282b/2
  Product_00657/1 -> Divide_7282b/1
  State_i_gd_GFL_16_d36c8/1 -> Product_00657/2
  Constant_-1_dcf39/1 -> Product_78f6d/1
  Product_54992/1 -> Product_00657/1
  Power_f2671/1 -> Product_54992/2
  Constant_2.0_3aa63/1 -> Power_f2671/2
  Constant_Vbase_04f09/1 -> Power_f2671/1
  Product_78f6d/1 -> Product_c2651/1
  Constant_Lg_pu_f9c71/1 -> Product_54992/1
  Product_32ca2/1 -> Product_3b637/1
  Subtract_08bc4/1 -> Subtract_bba52/1
  Product_096f6/1 -> Subtract_08bc4/2
  Constant_Vdcbase_5e2db/1 -> Product_e5c80/2
  Subtract_2ca08/1 -> Product_6656f/2
  State_i_gd_GFL_16_cdb96/1 -> Product_54d20/2
  MathFunc_sin_8f628/1 -> Product_f25ba/2
  Input_v_q_GFL_16_384ed/1 -> Product_f25ba/1
  State_Phi_ga_GFL_16_f5490/1 -> Add_7ab97/2
  MathFunc_cos_41cff/1 -> Product_67394/2
  Product_04461/1 -> Product_37675/1
  Add_9b5ff/1 -> Add_c3ad8/1
  Product_93fff/1 -> Add_9b5ff/2
  Input_i_dc_GFL_16_33564/1 -> Product_547ce/2
  Product_76327/1 -> Add_761ef/2
  Subtract_89bff/1 -> Product_76327/2
  State_V_dc_GFL_16_5e24a/1 -> Subtract_89bff/1
  Constant_P_od_098ac/1 -> Product_76327/1
  Constant_Lg_pu_a2551/1 -> Product_78f6d/2
  Subtract_29b3a/1 -> Product_14e77/2
  State_Idv_GFL_16_247ed/1 -> Add_17370/2
  Product_14e77/1 -> Add_17370/1
  Product_cde4f/1 -> Subtract_29b3a/2
  MathFunc_sin_dc889/1 -> Product_cde4f/2
  State_theta_pll_GFL_16_4472e/1 -> MathFunc_sin_dc889/1
  Input_v_q_GFL_16_2d758/1 -> Product_cde4f/1
  Product_b3dfc/1 -> Subtract_29b3a/1
  State_i_gq_GFL_16_0cd26/1 -> Product_fc96c/2
  State_theta_pll_GFL_16_59dfe/1 -> MathFunc_cos_17176/1
  Input_v_d_GFL_16_6e82b/1 -> Product_b3dfc/1
  Constant_Vbase_191ea/1 -> Power_787dc/1
  Constant_Bva_8474d/1 -> Product_6d03d/2
  Constant_-1_eab2d/1 -> Product_6d03d/1
  Constant_P_id_f32f0/1 -> Product_93fff/1
  Divide_a3f2f/1 -> Add_9b5ff/1
  Product_fc96c/1 -> Divide_a3f2f/1
  Constant_2.0_facde/1 -> Power_787dc/2
  Product_54d20/1 -> Product_096f6/1
  Divide_9b77b/1 -> Subtract_08bc4/1
  Constant_Vdcbase_783e7/1 -> Divide_9b77b/2
  Product_c8d64/1 -> Product_547ce/1
  State_V_dc_GFL_16_d7b7a/1 -> Product_c8d64/2
  Constant_f0_33442/1 -> Product_04461/2
  Power_de356/1 -> Product_f9df0/2
  Constant_Vbase_af0bd/1 -> Power_de356/1
  Constant_2.0_3ec7d/1 -> Product_538c9/1

== system IEEE14_case/GFL_16/d_i_gd_GFL_16_block ==
  note: d_i_gd_GFL_16 in case14gfl
      | $\frac{2\,\pi \,\mathrm{Sbase}\,f_{0}\,\left(\Phi _{\mathrm{gb},\mathrm{GFL},16}+P_{\mathrm{id}}\,\left(\mathrm{Idv}_{\mathrm{GFL},16}+\Phi _{\mathrm{ga},\mathrm{GFL},16}-i_{\mathrm{gd},\mathrm{GFL},16}+P_{\mathrm{od}}\,\left(V_{\mathrm{dc},\mathrm{GFL},16}-\mathrm{Vdcbase}\,\mathrm{Vdc}_{\mathrm{ref}}\right)-\mathrm{Bva}\,\mathrm{Vbase}\,\left(v_{d,\mathrm{GFL},16}\,\cos\left(\theta _{\mathrm{pll},\mathrm{GFL},16}\right)-v_{q,\mathrm{GFL},16}\,\sin\left(\theta _{\mathrm{pll},\mathrm{GFL},16}\right)\right)\right)-\frac{\mathrm{Rg}_{\mathrm{pu}}\,{\mathrm{Vbase}}^2\,i_{\mathrm{gd},\mathrm{GFL},16}}{\mathrm{Sbase}}\right)}{\mathrm{Lg}_{\mathrm{pu}}\,{\mathrm{Vbase}}^2}$
      | Automatically generated on 2025-10-09 21:35:43 .
  Input_v_d_GFL_16_f719a : Inport
  State_theta_pll_GFL_16_0c1ff : Inport  Port=2
  Input_v_q_GFL_16_05df1 : Inport  Port=3
  State_theta_pll_GFL_16_7ef19 : Inport  Port=4
  State_Idv_GFL_16_f06d3 : Inport  Port=5
  State_V_dc_GFL_16_82701 : Inport  Port=6
  State_Phi_ga_GFL_16_0916f : Inport  Port=7
  State_i_gd_GFL_16_54b5c : Inport  Port=8
  State_Phi_gb_GFL_16_1e17f : Inport  Port=9
  State_i_gd_GFL_16_5edc7 : Inport  Port=10
  Add_4e632 : Sum
  Add_63c44 : Sum
  Add_88fd2 : Sum
  Add_ca7fb : Sum
  Constant_-1_6fe25 : Constant  Value=-1
  Constant_2.0_08800 : Constant  Value=2.0
  Constant_2.0_22e48 : Constant  Value=2.0
  Constant_2.0_5286a : Constant  Value=2.0
  Constant_Bva_b76c1 : Constant  Value=Bva
  Constant_Lg_pu_75523 : Constant  Value=Lg_pu
  Constant_P_id_8548c : Constant  Value=P_id
  Constant_P_od_03888 : Constant  Value=P_od
  Constant_Rg_pu_0424f : Constant  Value=Rg_pu
  Constant_Sbase_55b11 : Constant  Value=Sbase
  Constant_Sbase_8e537 : Constant  Value=Sbase
  Constant_Vbase_22d09 : Constant  Value=Vbase
  Constant_Vbase_4ba6d : Constant  Value=Vbase
  Constant_Vbase_d0e24 : Constant  Value=Vbase
  Constant_Vdc_ref_50fd9 : Constant  Value=Vdc_ref
  Constant_Vdcbase_e258e : Constant  Value=Vdcbase
  Constant_f0_35aba : Constant  Value=f0
  Constant_pi_8a19a : Constant  Value=pi
  Divide_40844 : Product  Inputs=*/
  Divide_64d79 : Product  Inputs=*/
  MathFunc_cos_80b22 : Trigonometry  Operator=cos
  MathFunc_sin_63ac3 : Trigonometry
  Power_9115f : Math  Operator=pow
  Power_f930b : Math  Operator=pow
  Product_2e615 : Product
  Product_3d397 : Product
  Product_659de : Product
  Product_6e6b3 : Product
  Product_7319b : Product
  Product_7f7f7 : Product
  Product_87e64 : Product
  Product_9b4f0 : Product
  Product_b4b68 : Product
  Product_c6417 : Product
  Product_ed317 : Product
  Product_ee78c : Product
  Product_effe7 : Product
  Product_f2592 : Product
  Product_fe184 : Product
  Subtract_12f4b : Sum  Inputs=+-
  Subtract_c0bcd : Sum  Inputs=+-
  Subtract_e8ebf : Sum  Inputs=+-
  Subtract_ecb0f : Sum  Inputs=+-
  Blockout_d_i_gd_GFL_16_c534c : Outport
  wires:
  Product_7319b/1 -> Product_2e615/1
  Constant_Bva_b76c1/1 -> Product_f2592/2
  State_theta_pll_GFL_16_0c1ff/1 -> MathFunc_cos_80b22/1
  State_Phi_ga_GFL_16_0916f/1 -> Add_88fd2/2
  State_theta_pll_GFL_16_7ef19/1 -> MathFunc_sin_63ac3/1
  Product_f2592/1 -> Product_9b4f0/1
  Constant_-1_6fe25/1 -> Product_f2592/1
  Input_v_d_GFL_16_f719a/1 -> Product_7f7f7/1
  State_Phi_gb_GFL_16_1e17f/1 -> Add_ca7fb/2
  MathFunc_cos_80b22/1 -> Product_7f7f7/2
  State_i_gd_GFL_16_54b5c/1 -> Subtract_e8ebf/2
  Product_659de/1 -> Subtract_c0bcd/2
  Input_v_q_GFL_16_05df1/1 -> Product_659de/1
  Constant_Vdcbase_e258e/1 -> Product_effe7/2
  MathFunc_sin_63ac3/1 -> Product_659de/2
  Constant_Vbase_22d09/1 -> Product_9b4f0/2
  Product_7f7f7/1 -> Subtract_c0bcd/1
  Constant_Vdc_ref_50fd9/1 -> Product_effe7/1
  Product_9b4f0/1 -> Product_87e64/1
  Subtract_c0bcd/1 -> Product_87e64/2
  State_V_dc_GFL_16_82701/1 -> Subtract_12f4b/1
  Product_2e615/1 -> Divide_64d79/1
  Product_effe7/1 -> Subtract_12f4b/2
  Product_87e64/1 -> Add_63c44/1
  Product_fe184/1 -> Divide_64d79/2
  State_Idv_GFL_16_f06d3/1 -> Add_63c44/2
  Constant_Sbase_8e537/1 -> Divide_40844/2
  Product_ee78c/1 -> Add_4e632/2
  Constant_P_od_03888/1 -> Product_ee78c/1
  Subtract_12f4b/1 -> Product_ee78c/2
  Constant_Sbase_55b11/1 -> Product_c6417/2
  Add_63c44/1 -> Add_4e632/1
  Constant_pi_8a19a/1 -> Product_3d397/2
  Add_4e632/1 -> Add_88fd2/1
  Constant_Vbase_4ba6d/1 -> Power_f930b/1
  Constant_2.0_5286a/1 -> Power_f930b/2
  Add_88fd2/1 -> Subtract_e8ebf/1
  Product_ed317/1 -> Product_b4b68/1
  Constant_Rg_pu_0424f/1 -> Product_ed317/1
  Power_f930b/1 -> Product_ed317/2
  Constant_2.0_22e48/1 -> Product_3d397/1
  Product_6e6b3/1 -> Add_ca7fb/1
  Constant_P_id_8548c/1 -> Product_6e6b3/1
  Subtract_e8ebf/1 -> Product_6e6b3/2
  State_i_gd_GFL_16_5edc7/1 -> Product_b4b68/2
  Product_3d397/1 -> Product_c6417/1
  Product_b4b68/1 -> Divide_40844/1
  Product_c6417/1 -> Product_7319b/1
  Constant_f0_35aba/1 -> Product_7319b/2
  Add_ca7fb/1 -> Subtract_ecb0f/1
  Divide_40844/1 -> Subtract_ecb0f/2
  Constant_2.0_08800/1 -> Power_9115f/2
  Constant_Vbase_d0e24/1 -> Power_9115f/1
  Subtract_ecb0f/1 -> Product_2e615/2
  Constant_Lg_pu_75523/1 -> Product_fe184/1
  Power_9115f/1 -> Product_fe184/2
  Divide_64d79/1 -> Blockout_d_i_gd_GFL_16_c534c/1
